simulink model "Zero_sequence_current_protection_automatic_reclosing"  (R2023a)
settings: Solver=VariableStepAuto  StartTime=0.0  StopTime=1  RelTol=1e-3
libraries: spsDistributedParametersLineLib x2, dspswit3 x2, spsThreePhaseVIMeasurementLib x2, spsSequenceAnalyzerLib x2, spsThreePhaseBreakerLib x2, spsThreePhaseSourceLib x2, spsMultimeterLib x1, spsThreePhaseFaultLib x1, sps_lib x1
settings Model: SimulationMode=accelerator  Creator=Lightrain  LastModifiedBy=Lightrain

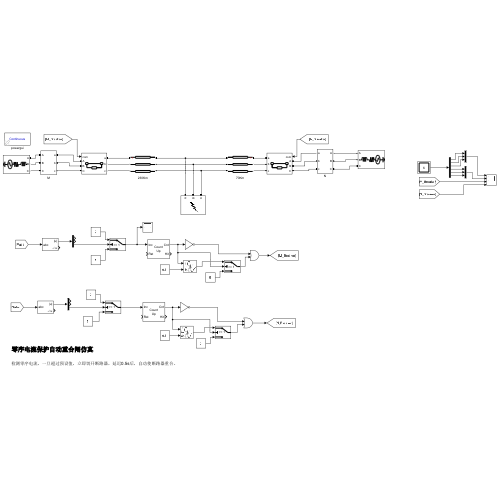
[thumbnail: Simulink's stored preview of the top-level diagram]
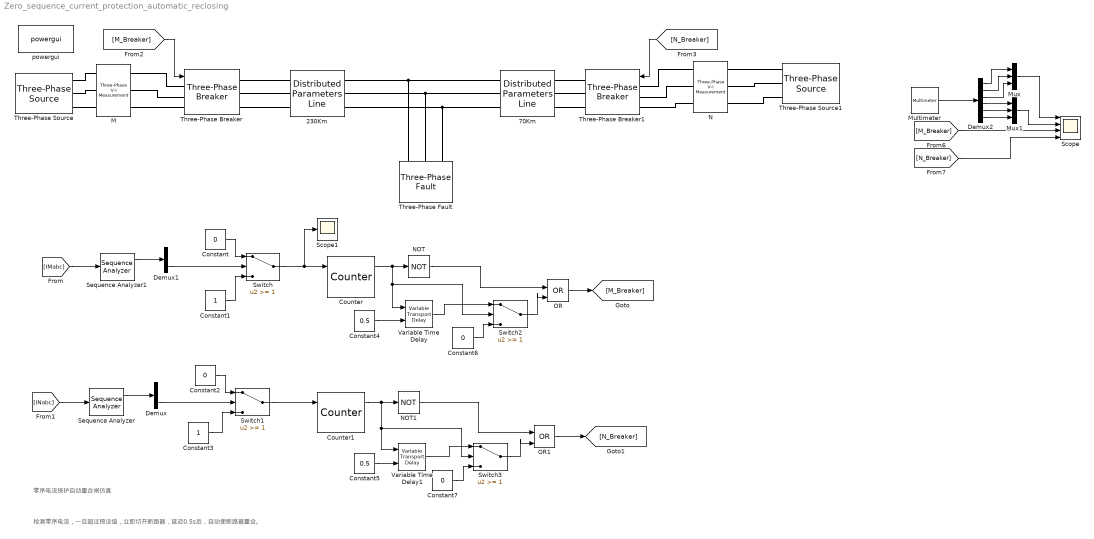
== system Zero_sequence_current_protection_automatic_reclosing ==
  note: 检测零序电流，一旦超过预设值，立即切开断路器，延迟0.5s后，自动使断路器重合。
  note: 零序电流保护自动重合闸仿真
  230Km : spsDistributedParametersLineLib/Distributed Parameters Line  Phases=3  Length=230  Frequency=60  Resistance=[0.01273 0.3864]  Inductance="[0.9337e-3  4.1264e-3]"  Capacitance=[12.74e-9 7.751e-9]  x1=[2.11879083924011e-10 501582.121364848 501582.121364848;314.159265358979 314.159265358979 314.159265358979;-1.70113795118969 0.273836781691284 -1.29695954510361]  x2=[2.54138273835604e-10 506371.691049996 506371.691049996;314.159265358979 314.159265358979 314.159265358979;2.50186070299399 0.273403807380817 -1.29739251941408]  x3=[1.2936022082018e-12 1862.20680522217 1862.20680522217;314.159265358979 314.159265358979 314.159265358979;2.21380525594337 0.110852392878641 -1.45994393391626]  x4=[1.87193540984712e-12 1862.49416354856 1862.49416354857;314.159265358979 314.159265358979 314.159265358979;-2.62293871898808 0.186492606615256 -1.38430372017964]  x5=0.00130074560409021  V1=[2.119e-10 5.016e+05 5.016e+05;314.2 314.2 314.2;-1.701 0.2738 -1.297]  V2=[2.541e-10 5.064e+05 5.064e+05;314.2 314.2 314.2;2.502 0.2734 -1.297]  I1=[1.294e-12 1862 1862;314.2 314.2 314.2;2.214 0.1109 -1.46]  I2=[1.872e-12 1862 1862;314.2 314.2 314.2;-2.623 0.1865 -1.384]  nHarmo=1  Measurements=None  Decoupling=off  VsMag0=0  VrMag0=0  VsAngle0=0  VrAngle0=0  IsMag0=0  IrMag0=0  IsAngle0=0  IrAngle0=0
      settings: LibrarySourceBlock=sps_lib/Power Grid Elements/Distributed Parameters Line
  70Km : spsDistributedParametersLineLib/Distributed Parameters Line  Phases=3  Length=70  Frequency=60  Resistance=[0.01273 0.3864]  Inductance="[0.9337e-3  4.1264e-3]"  Capacitance=[12.74e-9 7.751e-9]  x1=[1.34162029386686e-10 501581.934501311 501581.934501312;314.159265358979 314.159265358979 314.159265358979;-0.832995358379814 0.447198198676987 -1.12359812811791]  x2=[2.54138273835604e-10 506371.691049996 506371.691049996;314.159265358979 314.159265358979 314.159265358979;2.78613290014175 0.446767539894209 -1.12402878690069]  x3=[4.91827451910963e-12 1872.42766283359 1872.42766283358;314.159265358979 314.159265358979 314.159265358979;1.01322707211112 0.284493586275699 -1.28630274051921]  x4=[1.90046204097372e-12 1873.30482199933 1873.30482199934;314.159265358979 314.159265358979 314.159265358979;2.95846774462193 0.533502413677279 -1.03729391311761]  x5=0.00039587909689702  V1=[1.342e-10 5.016e+05 5.016e+05;314.2 314.2 314.2;-0.833 0.4472 -1.124]  V2=[2.541e-10 5.064e+05 5.064e+05;314.2 314.2 314.2;2.786 0.4468 -1.124]  I1=[4.918e-12 1872 1872;314.2 314.2 314.2;1.013 0.2845 -1.286]  I2=[1.9e-12 1873 1873;314.2 314.2 314.2;2.958 0.5335 -1.037]  nHarmo=1  Measurements=None  Decoupling=off  VsMag0=0  VrMag0=0  VsAngle0=0  VrAngle0=0  IsMag0=0  IrMag0=0  IsAngle0=0  IrAngle0=0
      settings: LibrarySourceBlock=sps_lib/Power Grid Elements/Distributed Parameters Line
  Constant{,2,6..7} (4 alike) : Constant  Value=0
  Constant1 : Constant
  Constant3 : Constant
  Constant4 : Constant  Value=0.5
  Constant5 : Constant  Value=0.5
  Counter : dspswit3/Counter  Direction=Up  CountEvent=Falling edge  CounterSize=User defined  MaxCount=255  InitialCount=0  Output=Count and Hit  HitValue=32  ResetInput=on  SamplesPerFrame=1  Ts=1  CntDtype=double  HitDtype=Logical
  Counter1 : dspswit3/Counter  Direction=Up  CountEvent=Falling edge  CounterSize=User defined  MaxCount=255  InitialCount=0  Output=Count and Hit  HitValue=32  ResetInput=on  SamplesPerFrame=1  Ts=1  CntDtype=double  HitDtype=Logical
  Demux : Demux  Outputs=3
  Demux1 : Demux  Outputs=3
  Demux2 : Demux  Outputs=6
  M : spsThreePhaseVIMeasurementLib/Three-Phase V-I Measurement  VoltageMeasurement=phase-to-ground  SetLabelV=on  LabelV=VMabc  Vpu=off  VpuLL=off  CurrentMeasurement=yes  SetLabelI=on  LabelI=IMabc  Ipu=off  Pbase=100e6  Vbase=500e3  OutputType=Complex  PhasorSimulation=off  PSBequivalent=0
  Multimeter : spsMultimeterLib/Multimeter  L=6  sel=[1 2 3 4 5 6]  yselected={}  Gain=[1 1 1 1 1 1]  OutputType=Complex  PlotAtSimulationStop=on  PhasorSimulation=off
  Mux : Mux  Inputs=3
  Mux1 : Mux  Inputs=3
  N : spsThreePhaseVIMeasurementLib/Three-Phase V-I Measurement  VoltageMeasurement=phase-to-ground  SetLabelV=on  LabelV=VNabc  Vpu=off  VpuLL=off  CurrentMeasurement=yes  SetLabelI=on  LabelI=INabc  Ipu=off  Pbase=100e6  Vbase=500e3  OutputType=Complex  PhasorSimulation=off  PSBequivalent=0
  NOT : Logic  Operator=NOT  IconShape=distinctive  AllPortsSameDT=off  OutDataTypeStr=boolean
  NOT1 : Logic  Operator=NOT  IconShape=distinctive  AllPortsSameDT=off  OutDataTypeStr=boolean
  OR : Logic  Operator=OR  IconShape=distinctive  AllPortsSameDT=off  OutDataTypeStr=boolean
  OR1 : Logic  Operator=OR  IconShape=distinctive  AllPortsSameDT=off  OutDataTypeStr=boolean
  Scope : Scope  NumInputPorts=4
  Scope1 : Scope
  Sequence Analyzer : spsSequenceAnalyzerLib/Sequence Analyzer  Freq=60  n=1  seq=Positive Negative Zero  InInit=[1, 0]  Ts=0
      settings: LibrarySourceBlock=sps_lib/Sensors and Measurements/Sequence Analyzer
  Sequence Analyzer1 : spsSequenceAnalyzerLib/Sequence Analyzer  Freq=60  n=1  seq=Positive Negative Zero  InInit=[1, 0]  Ts=0
      settings: LibrarySourceBlock=sps_lib/Sensors and Measurements/Sequence Analyzer
  Switch{,1..3} (4 alike) : Switch  Threshold=1  SaturateOnIntegerOverflow=off  InputSameDT=off
  Three-Phase Breaker : spsThreePhaseBreakerLib/Three-Phase Breaker  InitialState=closed  SwitchA=on  SwitchB=on  SwitchC=on  SwitchTimes="[1/60  5/60]"  External=on  BreakerResistance=0.01  SnubberResistance=1e6  SnubberCapacitance=inf  Measurements=None
  Three-Phase Breaker1 : spsThreePhaseBreakerLib/Three-Phase Breaker  InitialState=closed  SwitchA=on  SwitchB=on  SwitchC=on  SwitchTimes="[1/60  5/60]"  External=on  BreakerResistance=0.01  SnubberResistance=1e6  SnubberCapacitance=inf  Measurements=None
  Three-Phase Fault : spsThreePhaseFaultLib/Three-Phase Fault  InitialStates=0  FaultA=on  FaultB=off  FaultC=off  GroundFault=on  SwitchTimes=[0.2 0.3]  External=off  SwitchStatus=NaN  FaultResistance=0.001  GroundResistance=0.01  SnubberResistance=1e6  SnubberCapacitance=inf  Measurements=Fault voltages and currents
  Three-Phase Source : spsThreePhaseSourceLib/Three-Phase Source  InternalConnection=Yg  VoltagePhases=off  Voltage=500e3  PhaseAngle=0  Voltage_phases=[25e3 25e3 25e3]/sqrt(3)  PhaseAngles_phases=[0 -120 +120]  Frequency=50  NonIdealSource=on  SpecifyImpedance=off  Resistance=0.8929  Inductance=16.58e-3  ShortCircuitLevel=100e6  BaseVoltage=25e3  XRratio=7  BusType=swing  Pref=10e3  Qref=0  Prefabc=[10e3, 10e3, 10e3]  Qrefabc=[0, 0, 0]  Qmin=-inf  Qmax=inf
  Three-Phase Source1 : spsThreePhaseSourceLib/Three-Phase Source  InternalConnection=Yg  VoltagePhases=off  Voltage=500e3  PhaseAngle=0  Voltage_phases=[25e3 25e3 25e3]/sqrt(3)  PhaseAngles_phases=[0 -120 +120]  Frequency=50  NonIdealSource=on  SpecifyImpedance=off  Resistance=0.8929  Inductance=16.58e-3  ShortCircuitLevel=100e6  BaseVoltage=25e3  XRratio=7  BusType=swing  Pref=10e3  Qref=0  Prefabc=[10e3, 10e3, 10e3]  Qrefabc=[0, 0, 0]  Qmin=-inf  Qmax=inf
  Variable Time Delay : VariableTransportDelay  MaximumDelay=10
  Variable Time Delay1 : VariableTransportDelay  MaximumDelay=10
  powergui : sps_lib/powergui  Priority=1  SimulationMode=Continuous  SampleTime=50e-6  frequency=60  Iterations=50  frequencyindice=60  Pbase=100e6  ErrMax=1e-4  UnitsV=kV  UnitsW=MW  buscounter=0  FunctionMessages=off  echomessages=off  EnableUseOfTLC=off  CurrentSourceSwitches=off  DisableSnubberDevices=off  DisableRonSwitches=off  DisableVfSwitches=off  DisplayEquations=off  AutomaticDiscreteSolvers=off  SolverType=Tustin/Backward Euler (TBE)  Interpol=off  ExternalGateDelay=off  methode=off  Ts=100  x0status=blocks  SPID=on  SwTol=0  HookPort=off  NonlinearTolerance=1e-4  nMaxIteration=100  ContinueOnMaxIteration=off  RestoreLinks=warning  ResistiveCurrentMeasurement=off  Frange=[0:2:500]  Ylog=off  Xlog=on  ShowGrid=off  save=off  variable=ZData  structure=0  ZoomFFT=off  StartTime=0.0  cycles=1  DisplayStyle=1  fundamental=60  FreqAxis=off  MaxFrequency=1000  frequencyindicesteady=1  RmsSteady=1  display=off
  wires:
  Sequence Analyzer/1 -> Demux/1
  Sequence Analyzer1/1 -> Demux1/1
  [IMabc] -> Sequence Analyzer1/1
  [INabc] -> Sequence Analyzer/1
  Constant/1 -> Switch/1
  Constant1/1 -> Switch/3
  Switch/1 -> Scope1/1, Counter/1
  Counter/1 -> Switch2/2, Variable Time Delay/1, NOT/1
  Counter1/1 -> NOT1/1, Switch3/2, Variable Time Delay1/1
  Constant2/1 -> Switch1/1
  Constant3/1 -> Switch1/3
  Switch1/1 -> Counter1/1
  [M_Breaker] -> Three-Phase Breaker/1
  [N_Breaker] -> Three-Phase Breaker1/1
  Constant4/1 -> Variable Time Delay/2
  NOT/1 -> OR/1
  OR/1 -> [M_Breaker]
  Constant5/1 -> Variable Time Delay1/2
  NOT1/1 -> OR1/1
  OR1/1 -> [N_Breaker]
  Variable Time Delay/1 -> Switch2/1
  Constant6/1 -> Switch2/3
  Switch2/1 -> OR/2
  Variable Time Delay1/1 -> Switch3/1
  Constant7/1 -> Switch3/3
  Switch3/1 -> OR1/2
  Demux1/3 -> Switch/2
  Demux/3 -> Switch1/2
  [M_Breaker] -> Scope/3
  [N_Breaker] -> Scope/4
  Multimeter/1 -> Demux2/1
  Mux/1 -> Scope/1
  Demux2/1 -> Mux/1
  Demux2/2 -> Mux/2
  Demux2/3 -> Mux/3
  Demux2/4 -> Mux1/1
  Demux2/5 -> Mux1/2
  Demux2/6 -> Mux1/3
  Mux1/1 -> Scope/2
  connections:
  Three-Phase Source/RConn1 -- M/LConn1
  Three-Phase Source/RConn2 -- M/LConn2
  Three-Phase Source/RConn3 -- M/LConn3
  Three-Phase Fault/LConn1 -- 70Km/RConn1 -- 230Km/RConn1
  Three-Phase Fault/LConn2 -- 70Km/RConn2 -- 230Km/RConn2
  Three-Phase Fault/LConn3 -- 70Km/RConn3 -- 230Km/RConn3
  M/RConn3 -- Three-Phase Breaker/LConn3
  M/RConn2 -- Three-Phase Breaker/LConn2
  M/RConn1 -- Three-Phase Breaker/LConn1
  Three-Phase Breaker/RConn1 -- 230Km/LConn1
  Three-Phase Breaker/RConn2 -- 230Km/LConn2
  Three-Phase Breaker/RConn3 -- 230Km/LConn3
  N/LConn3 -- Three-Phase Source1/RConn3
  N/LConn2 -- Three-Phase Source1/RConn2
  N/LConn1 -- Three-Phase Source1/RConn1
  Three-Phase Breaker1/LConn1 -- N/RConn1
  Three-Phase Breaker1/LConn2 -- N/RConn2
  Three-Phase Breaker1/LConn3 -- N/RConn3
  70Km/LConn1 -- Three-Phase Breaker1/RConn1
  70Km/LConn2 -- Three-Phase Breaker1/RConn2
  70Km/LConn3 -- Three-Phase Breaker1/RConn3
